simulink model "SoftPwmOutputDemo"  (R2017a)
settings: Solver=FixedStepAuto  StartTime=0.0  StopTime=20  RelTol=1e-3  EnableMultiTasking=on
undefined symbols (not defined in the file or in its folder): Rec, SDTV, strel
libraries: simulink x4, visionstatistics x1, visionconversions x1, visionmorphops x1, embdlinuxlib x1
settings Model: SimulationMode=external  Creator=Shogo  LastModifiedBy=Shogo
settings SolverCC: PositivePriorityOrder=on
settings OptimizationCC: LifeSpan=1  MaxStackSize=64
settings DebuggingCC: ParameterPrecisionLossMsg=none  SFUnexpectedBacktrackingDiag=warning  SFNoUnconditionalDefaultTransitionDiag=warning  SFExecutionAtInitializationDiag=none
settings HardwareCC: ProdBitPerPointer=32  ProdBitPerSizeT=32  ProdBitPerPtrDiffT=32  ProdLargestAtomicInteger=Long  ProdLargestAtomicFloat=Double  ProdWordSize=32  ProdHWDeviceType=ARM Compatible->ARM Cortex  UseEmbeddedCoderFeatures=off  UseSimulinkCoderFeatures=off
settings RTWCC: SystemTargetFile=ert.tlc  HardwareBoard=Raspberry Pi  TLCOptions=-aInlineSetEventsForThisBaseRateFcn=TLC_FALSE -aSuppressMultiTaskScheduler=TLC_FALSE -aRateBasedStepFcn=0  TemplateMakefile=ert_default_tmf  Description=Embedded Coder  RTWVerbose=off  Toolchain=GNU GCC Raspberry Pi
settings CodeAppCC: ForceParamTrailComments=on  OperatorAnnotations=on  MangleLength=10  MATLABSourceComments=on
settings ERTTargetCC: MultiwordLength=2048  ERTCustomFileBanners=off  SupportContinuousTime=on  SupportNonInlinedSFcns=on  RemoveResetFunc=off  SupportVariableSizeSignals=on  ModelStepFunctionPrototypeControlCompliant=off  ExtMode=on  ExtModeMexArgs='192.168.11.13' 0 17725  ERTSrcFileBannerTemplate=codertarget_code_template.cgt  ERTHdrFileBannerTemplate=codertarget_code_template.cgt  ERTDataSrcFileTemplate=codertarget_code_template.cgt  ERTDataHdrFileTemplate=codertarget_code_template.cgt
settings ConfigComp: CovMetricSettings=dw  CovHtmlReporting=on  CovSaveCumulativeToWorkspaceVar=on  CovSaveSingleToWorkspaceVar=on  CovExternalEMLEnable=off

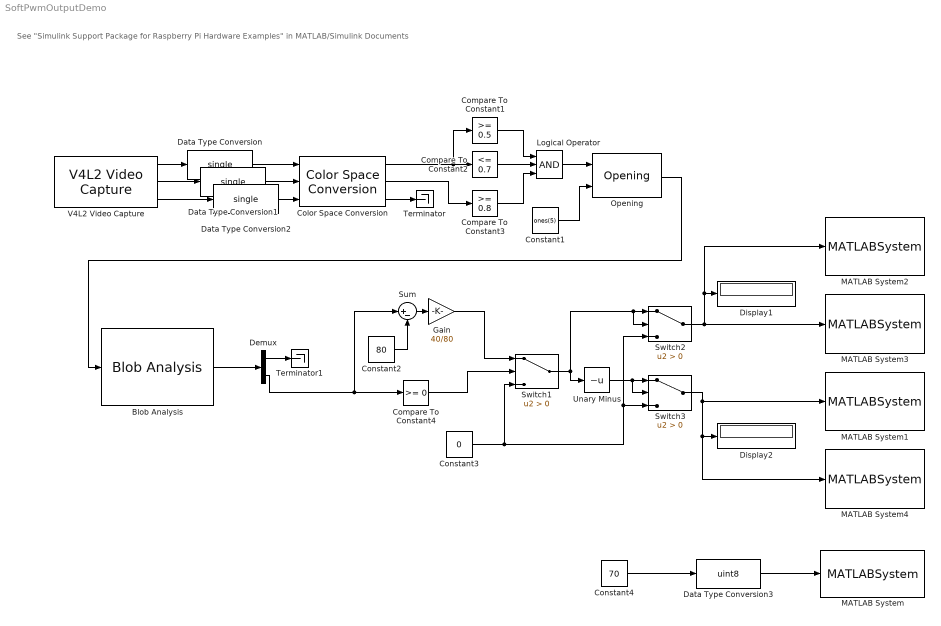
== system SoftPwmOutputDemo ==
  note: See "Simulink Support Package for Raspberry Pi Hardware Examples" in MATLAB/Simulink Documents
  Blob Analysis : visionstatistics/Blob Analysis  Tag=vipblks_row_conv  area=off  centroid=on  bBox=off  majorAxis=off  minorAxis=off  angle=off  eccentricity=off  equivDiameterSq=off  extent=off  perimeter=off  maxBlobs=1  warnIfNumBlobsExceeded=on  isCount=off  useMinArea=off  minArea=0  useMaxArea=off  maxArea=intmax('uint32')  excludeBorderBlob=off  outDT=double  isOutVarDim=off  isFill=on  fillValues=-1  conn=8  isLabel=off  outputMode=Binary point scaling  outputWordLength=32  outputFracLength=16  firstCoeffMode=Binary point scaling  firstCoeffWordLength=16  firstCoeffFracLength=14  secondCoeffMode=Binary point scaling  secondCoeffWordLength=32  secondCoeffFracLength=16  accumMode=Binary point scaling  accumWordLength=32  accumFracLength=0  prodOutputMode=Binary point scaling  prodOutputWordLength=32  prodOutputFracLength=16  roundingMode=Floor  overflowMode=off
      settings: SourceProductName=Computer Vision System Toolbox
  Color Space Conversion : visionconversions/Color Space  Conversion  conversion=Obsolete  conversionActive=R'G'B' to HSV  wp_str=D65  rec=Rec. 601 (SDTV)  sys=1125/60/2:1  imagePorts=Separate color signals
      settings: SourceProductName=Computer Vision System Toolbox
  Compare To Constant1 : simulink/Logic and Bit Operations/Compare To Constant  relop=>=  const=0.5  OutDataTypeStr=boolean
  Compare To Constant2 : simulink/Logic and Bit Operations/Compare To Constant  relop=<=  const=0.7  OutDataTypeStr=boolean
  Compare To Constant3 : simulink/Logic and Bit Operations/Compare To Constant  relop=>=  const=0.8  OutDataTypeStr=boolean
  Compare To Constant4 : simulink/Logic and Bit Operations/Compare To Constant  relop=>=  const=0  OutDataTypeStr=boolean
  Constant1 : Constant  Value=ones(5)  OutDataTypeStr=boolean
  Constant2 : Constant  Value=80  OutDataTypeStr=single
  Constant3 : Constant  Value=0  OutDataTypeStr=single
  Constant4 : Constant  Value=70  OutDataTypeStr=single
  Data Type Conversion : DataTypeConversion  OutDataTypeStr=single
  Data Type Conversion1 : DataTypeConversion  OutDataTypeStr=single
  Data Type Conversion2 : DataTypeConversion  OutDataTypeStr=single
  Data Type Conversion3 : DataTypeConversion  OutDataTypeStr=uint8
  Demux : Demux  Outputs=2
  Display1 : Display
  Display2 : Display
  Gain : Gain  Gain=40/80  OutDataTypeStr=double
  Logical Operator : Logic  Inputs=3  AllPortsSameDT=off  OutDataTypeStr=boolean
  MATLAB System : MATLABSystem  System=PwmOutput  Pin=18  Mode=0  Divisor=375  Range=1024
      mask Type: PwmOutput
      mask Display:
      | disp('PWM Write (18)');
      | port_label('input',1,'u');
  MATLAB System1 : MATLABSystem  System=SoftPwmOutput  Pin=19  InitialValue=0  PwmRange=100
      mask Type: SoftPwmOutput
      mask Display:
      | disp('SoftPWM Write (19)');
      | port_label('input',1,'u');
  MATLAB System2 : MATLABSystem  System=SoftPwmOutput  Pin=20  InitialValue=0  PwmRange=100
      mask Type: SoftPwmOutput
      mask Display:
      | disp('SoftPWM Write (20)');
      | port_label('input',1,'u');
  MATLAB System3 : MATLABSystem  System=SoftPwmOutput  Pin=21  InitialValue=0  PwmRange=100
      mask Type: SoftPwmOutput
      mask Display:
      | disp('SoftPWM Write (21)');
      | port_label('input',1,'u');
  MATLAB System4 : MATLABSystem  System=SoftPwmOutput  Pin=26  InitialValue=0  PwmRange=100
      mask Type: SoftPwmOutput
      mask Display:
      | disp('SoftPWM Write (26)');
      | port_label('input',1,'u');
  Opening : visionmorphops/Opening  nhoodsrc=Input port  strel=strel('disk',5)
      settings: SourceProductName=Computer Vision System Toolbox  SourceProductBaseCode=VP
  Sum : Sum  Inputs=|+-
  Switch1 : Switch  Criteria=u2 > Threshold
  Switch2 : Switch  Criteria=u2 > Threshold  OutDataTypeStr=uint8
  Switch3 : Switch  Criteria=u2 > Threshold  OutDataTypeStr=uint8
  Terminator : Terminator
  Terminator1 : Terminator
  Unary Minus : UnaryMinus
  V4L2 Video Capture : embdlinuxlib/V4L2 Video Capture  m_devName='/dev/video0'  roi=[0, 0, 640, 480]  imSizeSelection=160x120  imSize=[640, 480]  pixelFormat=RGB  pixelOrder=Planar  sampleTime=1/10  simOutput=Colorbars  blockPlatform=Raspberry Pi
  wires:
  V4L2 Video Capture/1 -> Data Type Conversion/1
  V4L2 Video Capture/2 -> Data Type Conversion1/1
  V4L2 Video Capture/3 -> Data Type Conversion2/1
  Color Space Conversion/1 -> Compare To Constant2/1, Compare To Constant1/1
  Compare To Constant1/1 -> Logical Operator/1
  Compare To Constant2/1 -> Logical Operator/2
  Logical Operator/1 -> Opening/1
  Color Space Conversion/2 -> Compare To Constant3/1
  Color Space Conversion/3 -> Terminator/1
  Compare To Constant3/1 -> Logical Operator/3
  Blob Analysis/1 -> Demux/1
  Constant1/1 -> Opening/2
  Sum/1 -> Gain/1
  Constant2/1 -> Sum/2
  Compare To Constant4/1 -> Switch1/2
  Switch2/1 -> Display1/1, MATLAB System2/1, MATLAB System3/1
  Switch3/1 -> MATLAB System4/1, Display2/1, MATLAB System1/1
  Data Type Conversion/1 -> Color Space Conversion/1
  Data Type Conversion1/1 -> Color Space Conversion/2
  Data Type Conversion2/1 -> Color Space Conversion/3
  Demux/1 -> Terminator1/1
  Demux/2 -> Sum/1, Compare To Constant4/1
  Opening/1 -> Blob Analysis/1
  Unary Minus/1 -> Switch3/2, Switch3/1
  Switch1/1 -> Unary Minus/1, Switch2/2, Switch2/1
  Gain/1 -> Switch1/1
  Data Type Conversion3/1 -> MATLAB System/1
  Constant3/1 -> Switch1/3, Switch3/3, Switch2/3
  Constant4/1 -> Data Type Conversion3/1
